simulink model "WashingMachineControlSysytem"  (R2024b)
settings: Solver=VariableStepAuto  StartTime=0.0  StopTime=inf  RelTol=1e-3
settings Model: Creator=Thanu  LastModifiedBy=deepi

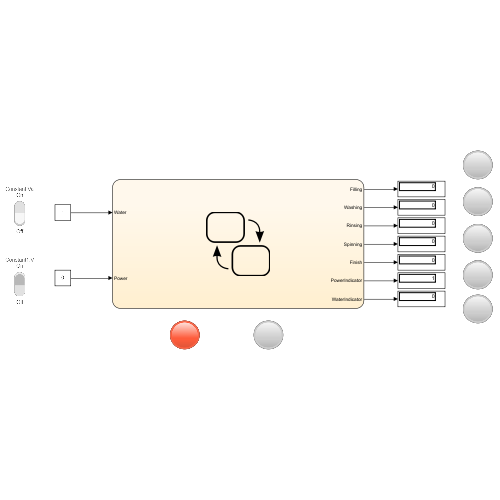
[thumbnail: Simulink's stored preview of the top-level diagram]
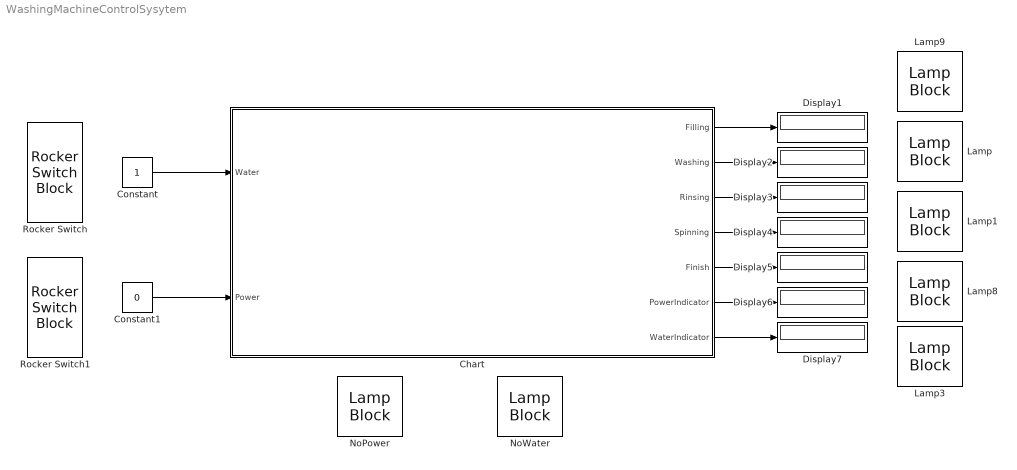
== system WashingMachineControlSysytem ==
  Chart : Stateflow chart  TreatAsAtomicUnit=on
  Constant : Constant
  Constant1 : Constant  Value=0
  Display{1..7} (7 alike) : Display
  Lamp{,1,3,8..9} (5 alike) : LampBlock  LabelPosition=Hide
  NoPower : LampBlock  LabelPosition=Hide
  NoWater : LampBlock  LabelPosition=Hide
  Rocker Switch : RockerSwitchBlock
      settings: Values={{'Off', 'On'}, [0 1]}
  Rocker Switch1 : RockerSwitchBlock
      settings: Values={{'Off', 'On'}, [0 1]}
  wires:
  Chart/7(WaterIndicator) -> Display7/1
  Chart/6(PowerIndicator) -> Display6/1
  Chart/1(Filling) -> Display1/1
  Chart/3(Rinsing) -> Display3/1
  Chart/2(Washing) -> Display2/1
  Chart/4(Spinning) -> Display4/1
  Chart/5(Finish) -> Display5/1
  Constant/1 -> Chart/1(Water)
  Constant1/1 -> Chart/2(Power)

== stateflow chart WashingMachineControlSysytem/Chart ==
  state Power_Supply
  state Water_Supply
  state Fill
    entry:
    Filling=1;
  state Wash
    entry:
    Filling=0,Washing=1;
  state Rinse
    entry:
    Washing=0,Rinsing=1;
  state Spin
    entry:
    Rinsing=0,Spinning=1;
  state End
    entry:
    Spinning=0,Finish=1
  state Power_indicator
    entry:
    PowerIndicator=1;
  state Water_Indicator
    entry:
    WaterIndicator=1;
  (default) -> Power_Supply
  Power_Supply -> Water_Supply [order 1] : [Power==1]
  Water_Supply -> Fill [order 1] : [Water==1]
  Fill -> Wash [order 1] : after(5,sec)
  Wash -> Rinse [order 1] : after(5,sec)
  Rinse -> Spin [order 1] : after(5,sec)
  Spin -> End [order 1] : after(2,sec)
  Spin -> Power_indicator [order 2] : [Power==0]
  Rinse -> Power_indicator [order 2] : [Power==0]
  Fill -> Power_indicator [order 2] : [Power==0]
  Power_Supply -> Power_indicator [order 2] : [Power==0]
  Wash -> Power_indicator [order 2] : [Power==0]
  Water_Supply -> Water_Indicator [order 2] : [Water==0]
  data: Water input; Power input; Filling output; Washing output; Rinsing output; Spinning output; Finish output; PowerIndicator output; WaterIndicator output
